simulink model "essaie_inversion"  (R2024b)
settings: Solver=VariableStepAuto  StartTime=0.0  StopTime=t_simu  RelTol=1e-3
values from neighbouring files (symbols this model uses):
  phi0 = -(R/(2*l))*(alpha_g_ini+alpha_d_ini)    (= 0)    [projet.m]
  x0 = 0    [projet.m]
  y0 = 0    [projet.m]
settings Model: Creator=yann  LastModifiedBy=yann

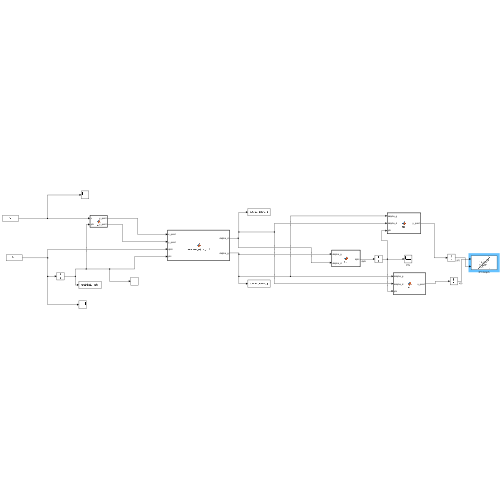
[thumbnail: Simulink's stored preview of the top-level diagram]
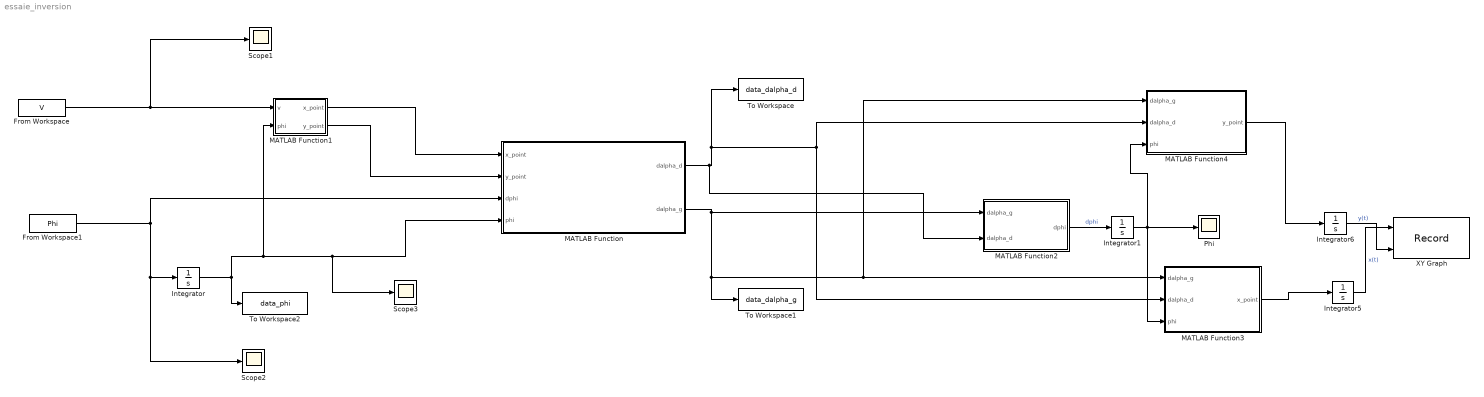
== system essaie_inversion ==
  From Workspace : FromWorkspace  VariableName=V
  From Workspace1 : FromWorkspace  VariableName=Phi
  Integrator : Integrator  InitialCondition=phi0
  Integrator1 : Integrator  InitialCondition=phi0
  Integrator5 : Integrator  InitialCondition=x0
  Integrator6 : Integrator  InitialCondition=y0
  MATLAB Function : MATLAB Function  TreatAsAtomicUnit=on
  MATLAB Function1 : MATLAB Function  TreatAsAtomicUnit=on
  MATLAB Function2 : MATLAB Function  TreatAsAtomicUnit=on
  MATLAB Function3 : MATLAB Function  TreatAsAtomicUnit=on
  MATLAB Function4 : MATLAB Function  TreatAsAtomicUnit=on
  Phi : Scope
  Scope1 : Scope
  Scope2 : Scope
  Scope3 : Scope
  To Workspace : ToWorkspace  VariableName=data_dalpha_d  SaveFormat=Timeseries  SampleTime=-1
  To Workspace1 : ToWorkspace  VariableName=data_dalpha_g  SaveFormat=Timeseries  SampleTime=-1
  To Workspace2 : ToWorkspace  VariableName=data_phi  SaveFormat=Timeseries  SampleTime=-1
  XY Graph : Record  FileSettingsInternal="{\"entries\":[{\"content\":{\"excelSettings\":{\"content\":{},\"type\":\"Streamout.ExcelSettings\"}},\"type\":\"Streamout.FileSettingStorage\",\"uuid\":\"\"}],\"packageUris\":[\"http:\\/\\/schema.mathworks.com\\/mf0\\/streamout_blocks\\/R2020a\"],\"version\":\"1.0\"}"  Layout=[1 1]  SignalsInternal="{\"entries\":[{\"content\":{\"signals\":[{\"content\":{\"blockPath\":[],\"dimensions\":[1],\"domain\":\"\",\"lineColor\":\"#a2142f\",\"plots\":[ 1 ],\"port\":1,\"sid\":[\"\"],\"signalID\":1,\"signalName\":\"x(t)\"},\"type\":\"RecordBlkView.Signal\",\"uuid\":\"\"},{\"content\":{\"blockPath\":[],\"dimensions\":[1],\"domain\":\"\",\"lineColor\":\"#139fff\",\"plots\":[ 1 ],\"port\":2,\"sid\":[\"\"],\"signalID\":2,\"signalName\":\"y(t)\"},\"type\":\"RecordBlkView.Signal\",\"uuid\":\"\"}]},\"type\":\"RecordBlkView.InputSignals\",\"uuid\":\"\"}],\"packageUris\":[\"http:\\/\\/schema.mathworks.com\\/mf0\\/streamout_blocks\\/R2020a\"],\"version\":\"1.0\"}"  VisualizationBindings="{\"xyplotplugin\":{\"info\":[{\"series\":[{\"bindingParametersList\":[{\"parameter\":\"X-Axis\",\"signalID\":1,\"signalName\":\"x(t)\"},{\"parameter\":\"Y-Axis\",\"signalID\":2,\"signalName\":\"y(t)\"}],\"seriesID\":0}],\"subplotID\":1}]}}"  CompatibilityTag=XY
  wires:
  From Workspace1/1 -> Scope2/1, Integrator/1, MATLAB Function/3(dphi)
  Integrator/1 -> To Workspace2/1, MATLAB Function1/2(phi), Scope3/1, MATLAB Function/4(phi)
  MATLAB Function/2(dalpha_g) -> MATLAB Function2/1(dalpha_g), MATLAB Function4/1(dalpha_g), MATLAB Function3/1(dalpha_g), To Workspace1/1
  MATLAB Function/1(dalpha_d) -> MATLAB Function2/2(dalpha_d), To Workspace/1, MATLAB Function4/2(dalpha_d), MATLAB Function3/2(dalpha_d)
  MATLAB Function1/1(x_point) -> MATLAB Function/1(x_point)
  MATLAB Function1/2(y_point) -> MATLAB Function/2(y_point)
  MATLAB Function4/1(y_point) -> Integrator6/1
  MATLAB Function3/1(x_point) -> Integrator5/1
  MATLAB Function2/1(dphi) -> Integrator1/1  "dphi"
  From Workspace/1 -> Scope1/1, MATLAB Function1/1(v)
  Integrator1/1 -> MATLAB Function3/3(phi), MATLAB Function4/3(phi), Phi/1
  Integrator5/1 -> XY Graph/1  "x(t)"
  Integrator6/1 -> XY Graph/2  "y(t)"

== matlab function essaie_inversion/MATLAB Function ==
  data: x_point input; dalpha_d output; y_point input; dphi input; phi input; dalpha_g output
function [dalpha_d, dalpha_g] = compute_alpha_dot(x_point, y_point, dphi, phi)
     v= (x_point^2 + y_point^2)^0.5;
     R=10e-2;
     l=15e-2;
     dalpha_g=(dphi*l + v)/R;
     dalpha_d=-2*(l*dphi)/R - dalpha_g;



end

== matlab function essaie_inversion/MATLAB Function1 ==
  data: v input; x_point output; phi input; y_point output
function [x_point,y_point] = fcn(v,phi)
    x_point=v*cos(phi);
    y_point=v*sin(phi);
end

== matlab function essaie_inversion/MATLAB Function2 ==
  data: dalpha_g input; dphi output; dalpha_d input
function dphi = fcn(dalpha_g, dalpha_d)
    R=10e-2;
    l=15e-2;
    

    dphi = (-R /(2*l)) *(dalpha_g+dalpha_d); 
end

== matlab function essaie_inversion/MATLAB Function3 ==
  data: dalpha_g input; x_point output; dalpha_d input; phi input
function x_point = fcn(dalpha_g,dalpha_d,phi)
    R=0.1;
    x_point = (R/2)*((dalpha_g+dalpha_d)*cos(phi)+(dalpha_d-dalpha_g)*sin(phi));
end

== matlab function essaie_inversion/MATLAB Function4 ==
  data: dalpha_g input; y_point output; dalpha_d input; phi input
function y_point = fcn(dalpha_g,dalpha_d,phi)
    R=0.1;
    y_point = (R/2)*((dalpha_g-dalpha_d)*cos(phi)+(dalpha_d+dalpha_g)*sin(phi));
end
